simulink model "PWM_PI"  (R2019b)
settings: Solver=ode23t  StartTime=0.0  StopTime=10e-3  MaxStep=1e-7  RelTol=1e-3  EnableMultiTasking=on
values from neighbouring files (symbols this model uses):
  Ap = wc*Tr    (= 0.861890988639)    [PWM_szab_init.m]
  fs = 20e3    (= 20000)    [PWM_szab_init.m]
  k_peak = 10    [PWM_szab_init.m]
  Ki = xref_n/Iki_n    (= 1)    [PWM_szab_init.m]
  L = 1e-3    (= 0.001)    [PWM_szab_init.m]
  R = 0.1    [PWM_szab_init.m]
  tau_Ki = 2e-6    (= 2e-06)    [PWM_szab_init.m]
  TI = 1/(wc*tan((pi/2-fi_t)*1/3))    [PWM_szab_init.m]
  U_dc = 150    [PWM_szab_init.m]
undefined symbols (not defined in the file or in its folder): sigbuilder_block
libraries: simulink x1
settings Model: Creator=Tálti  LastModifiedBy=kissd
settings DataIOCC: LimitDataPoints=on  SaveFormat=Array  ReturnWorkspaceOutputs=off
settings OptimizationCC: ExpressionDepthLimit=2147483647  LifeSpan=inf
settings DebuggingCC: UnderspecifiedInitializationDetection=Classic  MergeDetectMultiDrivingBlocksExec=none  SolverPrmCheckMsg=warning  StateNameClashWarn=warning  SFUnexpectedBacktrackingDiag=warning  SFNoUnconditionalDefaultTransitionDiag=warning  SFExecutionAtInitializationDiag=none  ArithmeticOperatorsInVariantConditions=warning
settings HardwareCC: ProdBitPerPointer=32  ProdBitPerSizeT=32  ProdBitPerPtrDiffT=32  ProdLargestAtomicFloat=None  ProdIntDivRoundTo=Undefined  ProdEndianess=Unspecified  ProdWordSize=32  ProdHWDeviceType=32-bit Generic
settings ModelReferenceCC: PropagateSignalLabelsOutOfModel=off
settings SFSimCC: SimUseLocalCustomCode=off  CustomCodeUndefinedFunction=UseInterfaceOnly
settings RTWCC: RTWUseLocalCustomCode=off
settings CodeAppCC: StateflowObjectComments=on
settings GRTTargetCC: TargetLangStandard=C89/C90 (ANSI)  GeneratePreprocessorConditionals=Disable all
settings ConfigComp: CovMetricSettings=dw  CovHtmlReporting=on  CovSaveCumulativeToWorkspaceVar=on  CovSaveSingleToWorkspaceVar=on  CovExternalEMLEnable=off

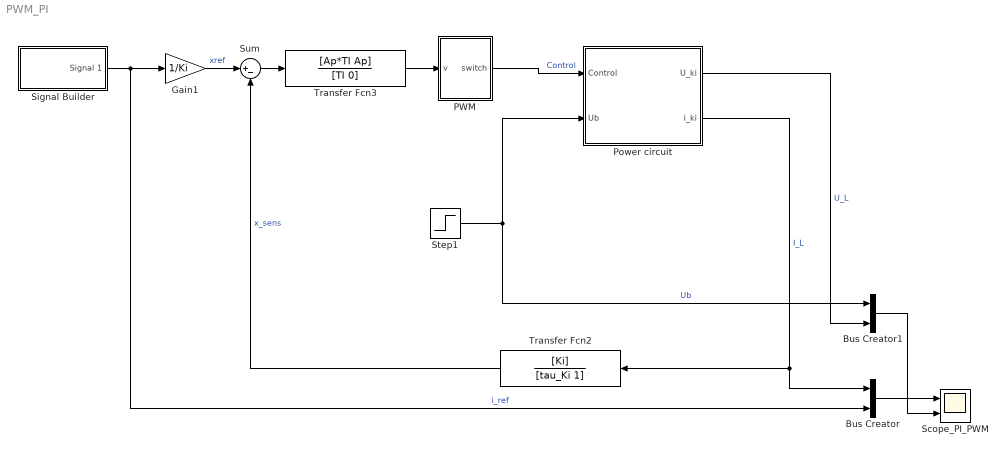
== system PWM_PI ==
  Bus Creator : BusCreator  Inputs=2
  Bus Creator1 : BusCreator  Inputs=2
  Gain1 : Gain  Gain=1/Ki
  PWM : Subsystem
  Power circuit : Subsystem
  Scope_PI_PWM : Scope  NumInputPorts=2
  Signal Builder : Subsystem  Tag=STV Subsys  LoadFcn=sigbuilder_block('load');  StartFcn=sigbuilder_block('start');  StopFcn=sigbuilder_block('stop');  ClipboardFcn=sigbuilder_block('clipboard');  mask(Sigbuilder block){tuvar=[0:10]}
      mask help: Simulink:masks:SigbuilderBlock_MD
      mask init:
      | if ~strcmp(get_param(bdroot(gcbh),'SimulationStatus'),'stopped') tuvar = sigbuilder_block('maskInit'); end
      settings: CopyFcn=sigbuilder_block('copy');  DeleteFcn=sigbuilder_block('delete');  ModelCloseFcn=sigbuilder_block('modelClose');  PreSaveFcn=sigbuilder_block('preSave');  PauseFcn=sigbuilder_block('pause');  ContinueFcn=sigbuilder_block('continue');  NameChangeFcn=sigbuilder_block('namechange');  OpenFcn=sigbuilder_block('open',[437.25 118.5 550.5 394.5 ]);  CloseFcn=sigbuilder_block('close');
      mask Display: plot(0, 0, 100, 100,[2, 2, 32, 32, 2], [68, 8, 8, 68, 68],[32, 2], [38, 38], [32, 19, 2],[53, 60, 44], [32, 17, 17, 2],[16, 16, 31, 31]);txt = getActiveGroup(gcbh);text(2, 100, txt,'verticalAlignment', 'top');
  Step1 : Step  Time=6e-3  Before=20  After=70  SampleTime=0
  Sum : Sum  Inputs=|+-
  Transfer Fcn2 : TransferFcn  Numerator=[Ki]  Denominator=[tau_Ki 1]
  Transfer Fcn3 : TransferFcn  Numerator=[Ap*TI Ap]  Denominator=[TI 0]
  wires:
  Signal Builder/1(Signal 1) -> Bus Creator/2, Gain1/1  "i_ref"
  Step1/1 -> Power circuit/2(Ub), Bus Creator1/1  "Ub"
  Bus Creator1/1 -> Scope_PI_PWM/2
  Bus Creator/1 -> Scope_PI_PWM/1
  Gain1/1 -> Sum/1  "xref"
  Transfer Fcn2/1 -> Sum/2  "x_sens"
  Sum/1 -> Transfer Fcn3/1
  Transfer Fcn3/1 -> PWM/1(v)
  Power circuit/2(i_ki) -> Bus Creator/1, Transfer Fcn2/1  "I_L"
  PWM/1(switch) -> Power circuit/1(Control)  "Control"
  Power circuit/1(U_ki) -> Bus Creator1/2  "U_L"

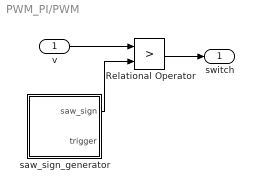
== system PWM_PI/PWM ==
  v : Inport
  Relational Operator : RelationalOperator  Operator=>  OutDataTypeStr=boolean  ZeroCross=off  RndMeth=Nearest
  saw_sign_generator : Subsystem
  switch : Outport  VectorParamsAs1DForOutWhenUnconnected=off
  wires:
  Relational Operator/1 -> switch/1
  v/1 -> Relational Operator/1
  saw_sign_generator/1(saw_sign) -> Relational Operator/2

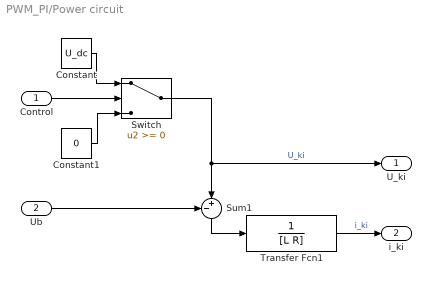
== system PWM_PI/Power circuit ==
  Control : Inport
  Ub : Inport  Port=2
  Constant : Constant  Value=U_dc
  Constant1 : Constant  Value=0
  Sum1 : Sum  Inputs=-+|
  Switch : Switch  ZeroCross=off
  Transfer Fcn1 : TransferFcn  Denominator=[L R]
  U_ki : Outport  VectorParamsAs1DForOutWhenUnconnected=off
  i_ki : Outport  Port=2  VectorParamsAs1DForOutWhenUnconnected=off
  wires:
  Control/1 -> Switch/2
  Sum1/1 -> Transfer Fcn1/1
  Switch/1 -> U_ki/1, Sum1/2  "U_ki"
  Constant1/1 -> Switch/3
  Constant/1 -> Switch/1
  Ub/1 -> Sum1/1
  Transfer Fcn1/1 -> i_ki/1  "i_ki"

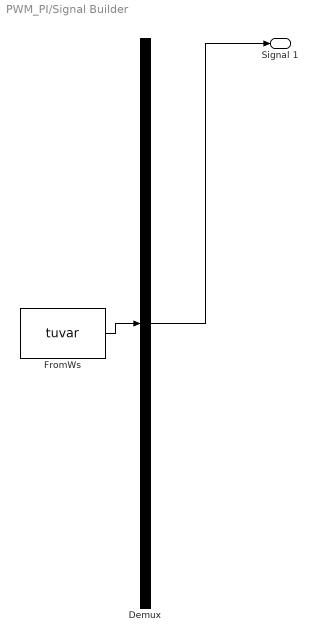
== system PWM_PI/Signal Builder ==
  Demux : Demux  Tag=STV Demux  Outputs=1
  FromWs : FromWorkspace  Tag=STV FromWs  VariableName=tuvar  SampleTime=0
      SigBuilderData=|
      | common.afterFinalStr = 'Extrapolate'
      | common.sampleTime = 0
      | dataSet.timeRange = [0 10]
      | dataSet.name = 'Group 1'
      | sbobj.Groups.Name = 'Group 1'
      | sbobj.Groups.Signals.Name = 'Signal 1'
      | sbobj.Groups.Signals.XData = [0 0.0001 0.00011 6 6 10]
      | sbobj.Groups.Signals.YData = [0 0 10 10 0 0]
  Signal 1 : Outport  Tag=STV Outport  VectorParamsAs1DForOutWhenUnconnected=off
  wires:
  Demux/1 -> Signal 1/1
  FromWs/1 -> Demux/1

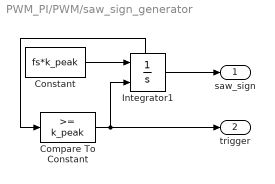
== system PWM_PI/PWM/saw_sign_generator ==
  Compare To Constant : simulink/Logic and Bit Operations/Compare To Constant  relop=>=  const=k_peak  OutDataTypeStr=boolean
  Constant : Constant  Value=fs*k_peak
  Integrator1 : Integrator  ExternalReset=rising  ShowStatePort=on
  saw_sign : Outport  VectorParamsAs1DForOutWhenUnconnected=off
  trigger : Outport  Port=2  VectorParamsAs1DForOutWhenUnconnected=off
  wires:
  Integrator1/1 -> saw_sign/1
  Integrator1/State -> Compare To Constant/1
  Constant/1 -> Integrator1/1
  Compare To Constant/1 -> trigger/1, Integrator1/2
